simulink model "lab6"  (R2023b)
settings: Solver=VariableStepAuto  StartTime=0.0  StopTime=10.0  RelTol=1e-3
settings Model: Creator=Spedrik Webster  LastModifiedBy=Spedrik Webster

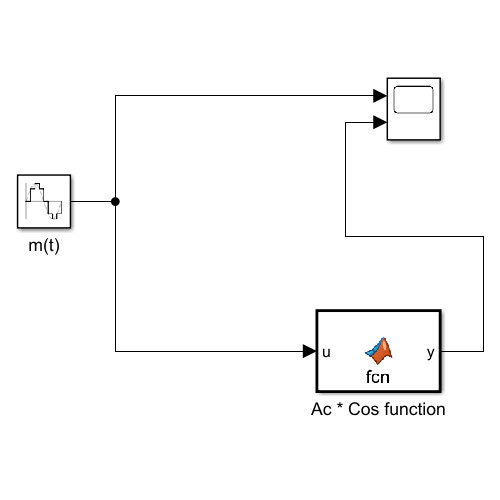
[thumbnail: Simulink's stored preview of the top-level diagram]
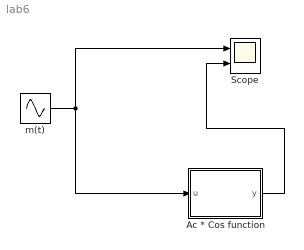
== system lab6 ==
  Ac * Cos function : MATLAB Function  TreatAsAtomicUnit=on
  Scope : Scope  NumInputPorts=2
  m(t) : Sin  Amplitude=2  Frequency=0.8  SampleTime=1/5000
  wires:
  m(t)/1 -> Ac * Cos function/1(u), Scope/1
  Ac * Cos function/1(y) -> Scope/2

== matlab function lab6/Ac * Cos function ==
  data: u input; y output
function y = fcn(u)
    var Ac 
    var kf
    var fc
    kf = 2 * pi;
    fc = 12;
    Ac = 5 * pi;
    y = Ac * cos((kf * u) + fc);
end
